simulink model "ex7_6_para"  (R2019b)
settings: Solver=VariableStepAuto  StartTime=0.0  StopTime=10.0  RelTol=1e-3
undefined symbols (not defined in the file): k
settings Model: Creator=Russty  LastModifiedBy=TimRo
settings DataIOCC: ReturnWorkspaceOutputs=off
settings DebuggingCC: ArithmeticOperatorsInVariantConditions=warning
settings SFSimCC: CustomCodeUndefinedFunction=UseInterfaceOnly

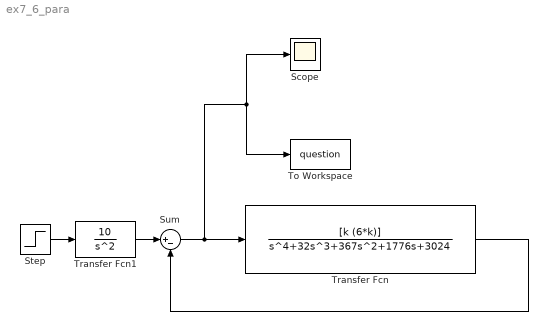
== system ex7_6_para ==
  Scope : Scope
  Step : Step  Time=0  SampleTime=0.001
  Sum : Sum  Inputs=|+-
  To Workspace : ToWorkspace  VariableName=question  SaveFormat=Timeseries  SampleTime=-1
  Transfer Fcn : TransferFcn  Numerator=[k (6*k)]  Denominator=[1 32 367 1776 3024]
  Transfer Fcn1 : TransferFcn  Numerator=[10]  Denominator=[1 0 0]
  wires:
  Transfer Fcn/1 -> Sum/2
  Sum/1 -> Transfer Fcn/1, To Workspace/1, Scope/1
  Step/1 -> Transfer Fcn1/1
  Transfer Fcn1/1 -> Sum/1
